simulink model "BBC"  (R2022b)
settings: Solver=VariableStepAuto  StartTime=0.0  StopTime=1  RelTol=1e-3
undefined symbols (not defined in the file): dct, dEv, Ev, sigbuilder_block
libraries: spsSeriesRLCBranchLib x3, spsVoltageMeasurementLib x2, spsControlledVoltageSourceLib x1, spsDiodeLib x1, fuzblock x1, spsGroundLib x1, spsCurrentMeasurementLib x1, spsMosfetLib x1, simulink x1, spspowerguiLib x1
settings Model: Creator=Dopechuro  LastModifiedBy=Dopechuro

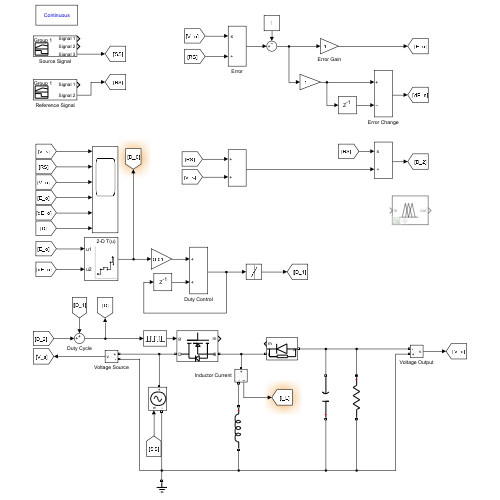
[thumbnail: Simulink's stored preview of the top-level diagram]
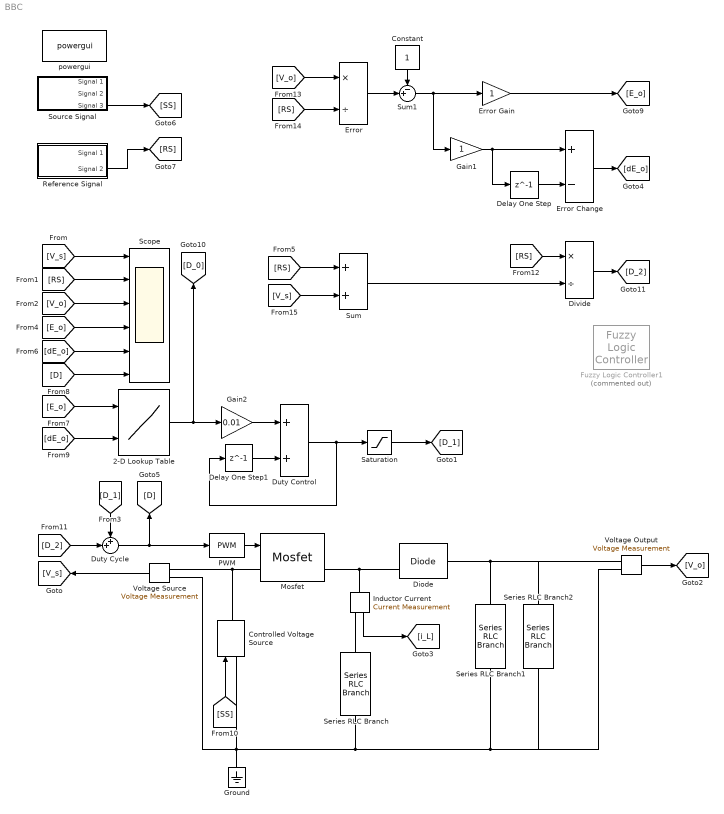
== system BBC ==
  2-D Lookup Table : Lookup_n-D  LookupTableObject=''  BreakpointsForDimension1=Ev  BreakpointsForDimension2=dEv  BreakpointsForDimension1FirstPoint=10  BreakpointsForDimension2FirstPoint=10  BreakpointsForDimension1Spacing=12  BreakpointsForDimension2Spacing=12  IndexSearchMethod=Evenly spaced points  Table=dct  InterpMethod=Nearest  DiagnosticForOutOfRangeInput=Warning  InternalRulePriority=Speed  OutDataTypeStr=Inherit: Inherit from 'Table data'  RndMeth=Simplest
      settings: InputPortMap=u0,u1
  Constant : Constant
  Controlled Voltage Source : spsControlledVoltageSourceLib/Controlled Voltage Source  Initialize=off  Source_Type=DC  Amplitude=0  Phase=0  Frequency=0  Measurements=None
  Delay One Step : Delay  DelayLength=1
  Delay One Step1 : Delay  DelayLength=1
  Diode : spsDiodeLib/Diode  Ron=0.001  Lon=0  Vf=0.8  IC=0  UseSnubber=0  Rs=500  Cs=250e-9  Measurements=on
  Divide : Product  Inputs=*/
  Duty Control : Sum
  Duty Cycle : Sum  Inputs=++|
  Error : Product  Inputs=*/
  Error Change : Sum  Inputs=+-
  Error Gain : Gain
  Fuzzy Logic Controller1 : fuzblock/Fuzzy Logic  Controller  Commented=on  FIS=bbFIS  OutputSampleNumber=101  DataType=double  FuzzifiedInputs=off  RuleFiringStrengths=off  RuleOutputs=off  AggregatedOutputs=off  SimulateUsing=Interpreted execution  OutOfRangeInputValueMessage=warning  NoRuleFiredMessage=warning  EmptyOutputFuzzySetMessage=warning
  Gain1 : Gain
  Gain2 : Gain  Gain=0.01
  Ground : spsGroundLib/Ground  LConnTagsString=a
  Inductor Current : spsCurrentMeasurementLib/Current Measurement  PhasorSimulation=off  OutputType=Complex  PSBequivalent=0
  Mosfet : spsMosfetLib/Mosfet  Ron=0.1  Lon=0  Rd=0.01  Vfd=0  IC=0  Rs=1e5  Cs=inf  Measurements=on
  PWM : simulink/Discontinuities/PWM  DisableCoverage=on  Period=1/1e5  InitialDelay=0  DisallowZeroDutyCycle=off  RunAtFixedTimeIntervals=off  SampleTime=0.1
  Reference Signal : Subsystem  Tag=STV Subsys  LoadFcn=sigbuilder_block('load');  StartFcn=sigbuilder_block('start');  StopFcn=sigbuilder_block('stop');  ClipboardFcn=sigbuilder_block('clipboard');  mask(Sigbuilder block){tuvar=[0:10]}
      mask help: Simulink:masks:SigbuilderBlock_MD
      mask init:
      | if ~strcmp(get_param(bdroot(gcbh),'SimulationStatus'),'stopped') tuvar = sigbuilder_block('maskInit'); end
      settings: CopyFcn=sigbuilder_block('copy');  DeleteFcn=sigbuilder_block('delete');  ModelCloseFcn=sigbuilder_block('modelClose');  PreSaveFcn=sigbuilder_block('preSave');  PauseFcn=sigbuilder_block('pause');  ContinueFcn=sigbuilder_block('continue');  NameChangeFcn=sigbuilder_block('namechange');  OpenFcn=sigbuilder_block('open',[530.25 309.75 550.5 399.75 ]);  CloseFcn=sigbuilder_block('close');
      mask Display: plot(0, 0, 100, 100,[2, 2, 32, 32, 2], [68, 8, 8, 68, 68],[32, 2], [38, 38], [32, 19, 2],[53, 60, 44], [32, 17, 17, 2],[16, 16, 31, 31]);txt = getActiveGroup(gcbh);text(2, 100, txt,'verticalAlignment', 'top');
  Saturation : Saturate  UpperLimit=0.9  LowerLimit=0
  Scope : Scope  NumInputPorts=6
  Series RLC Branch : spsSeriesRLCBranchLib/Series RLC Branch  LConnTagsString=__new0  RConnTagsString=__new0  BranchType=L  Resistance=1  Inductance=20e-6  SetiL0=off  InitialCurrent=0  Capacitance=1e-6  Setx0=off  InitialVoltage=0  Measurements=None
  Series RLC Branch1 : spsSeriesRLCBranchLib/Series RLC Branch  LConnTagsString=__new0  RConnTagsString=__new0  BranchType=C  Resistance=1  Inductance=1e-3  SetiL0=off  InitialCurrent=0  Capacitance=80e-6  Setx0=off  InitialVoltage=0  Measurements=None
  Series RLC Branch2 : spsSeriesRLCBranchLib/Series RLC Branch  LConnTagsString=__new0  RConnTagsString=__new0  BranchType=R  Resistance=5  Inductance=1e-3  SetiL0=off  InitialCurrent=0  Capacitance=1e-6  Setx0=off  InitialVoltage=0  Measurements=None
  Source Signal : Subsystem  Tag=STV Subsys  LoadFcn=sigbuilder_block('load');  StartFcn=sigbuilder_block('start');  StopFcn=sigbuilder_block('stop');  ClipboardFcn=sigbuilder_block('clipboard');  mask(Sigbuilder block){tuvar=[0:10]}
      mask help: Simulink:masks:SigbuilderBlock_MD
      mask init:
      | if ~strcmp(get_param(bdroot(gcbh),'SimulationStatus'),'stopped') tuvar = sigbuilder_block('maskInit'); end
      settings: CopyFcn=sigbuilder_block('copy');  DeleteFcn=sigbuilder_block('delete');  ModelCloseFcn=sigbuilder_block('modelClose');  PreSaveFcn=sigbuilder_block('preSave');  PauseFcn=sigbuilder_block('pause');  ContinueFcn=sigbuilder_block('continue');  NameChangeFcn=sigbuilder_block('namechange');  OpenFcn=sigbuilder_block('open',[395.25 256.5 550.5 399.75 ]);  CloseFcn=sigbuilder_block('close');
      mask Display: plot(0, 0, 100, 100,[2, 2, 32, 32, 2], [68, 8, 8, 68, 68],[32, 2], [38, 38], [32, 19, 2],[53, 60, 44], [32, 17, 17, 2],[16, 16, 31, 31]);txt = getActiveGroup(gcbh);text(2, 100, txt,'verticalAlignment', 'top');
  Sum : Sum
  Sum1 : Sum  Inputs=-+|
  Voltage Output : spsVoltageMeasurementLib/Voltage Measurement  PhasorSimulation=off  OutputType=Complex  PSBequivalent=0
  Voltage Source : spsVoltageMeasurementLib/Voltage Measurement  PhasorSimulation=off  OutputType=Complex  PSBequivalent=0
  powergui : spspowerguiLib/powergui  Priority=1  SimulationMode=Continuous  SampleTime=50e-6  frequency=60  Iterations=50  frequencyindice=0  Pbase=100e6  ErrMax=1e-4  UnitsV=kV  UnitsW=MW  buscounter=0  FunctionMessages=off  echomessages=off  EnableUseOfTLC=off  CurrentSourceSwitches=off  DisableSnubberDevices=off  DisableRonSwitches=off  DisableVfSwitches=off  DisplayEquations=off  AutomaticDiscreteSolvers=off  SolverType=Tustin/Backward Euler (TBE)  Interpol=off  ExternalGateDelay=off  methode=off  Ts=100  x0status=blocks  SPID=on  SwTol=0  HookPort=off  NonlinearTolerance=1e-4  nMaxIteration=100  ContinueOnMaxIteration=off  RestoreLinks=warning  ResistiveCurrentMeasurement=off  Frange=[0:2:500]  Ylog=off  Xlog=on  ShowGrid=off  save=off  variable=ZData  structure=0  ZoomFFT=off  StartTime=0.0  cycles=1  DisplayStyle=1  fundamental=60  FreqAxis=off  MaxFrequency=1000  frequencyindicesteady=1  RmsSteady=1  display=off
  wires:
  Voltage Source/1 -> [V_s]
  Inductor Current/1 -> [i_L]
  Voltage Output/1 -> [V_o]
  PWM/1 -> Mosfet/1
  [V_s] -> Scope/1
  [RS] -> Scope/2
  [V_o] -> Scope/3
  Error Change/1 -> [dE_o]
  Delay One Step/1 -> Error Change/2
  [E_o] -> Scope/4
  [dE_o] -> Scope/5
  [D] -> Scope/6
  Duty Cycle/1 -> [D], PWM/1
  [SS] -> Controlled Voltage Source/1
  [D_2] -> Duty Cycle/2
  [V_o] -> Error/1
  [RS] -> Error/2
  Error/1 -> Sum1/2
  Constant/1 -> Sum1/1
  Sum1/1 -> Gain1/1, Error Gain/1
  Error Gain/1 -> [E_o]
  Gain1/1 -> Error Change/1, Delay One Step/1
  Gain2/1 -> Duty Control/1
  Delay One Step1/1 -> Duty Control/2
  Duty Control/1 -> Saturation/1, Delay One Step1/1
  [D_1] -> Duty Cycle/1
  Saturation/1 -> [D_1]
  2-D Lookup Table/1 -> Gain2/1, [D_0]
  [E_o] -> 2-D Lookup Table/1
  [dE_o] -> 2-D Lookup Table/2
  [RS] -> Sum/1
  [V_s] -> Sum/2
  Divide/1 -> [D_2]
  Sum/1 -> Divide/2
  [RS] -> Divide/1
  Reference Signal/2(Signal 2) -> [RS]
  Source Signal/3(Signal 3) -> [SS]
  connections:
  Mosfet/LConn1 -- Controlled Voltage Source/RConn1 -- Voltage Source/LConn1
  Mosfet/RConn1 -- Inductor Current/LConn1 -- Diode/RConn1
  Diode/LConn1 -- Voltage Output/LConn2 -- Series RLC Branch2/LConn1 -- Series RLC Branch1/RConn1
  Voltage Output/LConn1 -- Series RLC Branch2/RConn1 -- Series RLC Branch1/LConn1 -- Series RLC Branch/RConn1 -- Ground/LConn1 -- Controlled Voltage Source/LConn1 -- Voltage Source/LConn2
  Inductor Current/RConn1 -- Series RLC Branch/LConn1

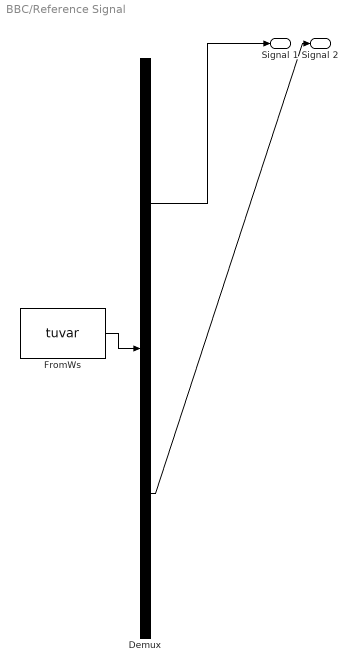
== system BBC/Reference Signal ==
  Demux : Demux  Tag=STV Demux  Outputs=2
      settings: DisplayOption=none
  FromWs : FromWorkspace  Tag=STV FromWs  VariableName=tuvar
      SigBuilderData=|
      | common.afterFinalStr = 'Extrapolate'
      | common.sampleTime = 0
      | dataSet.timeRange = [0 1]
      | dataSet.name = 'Group 1'
      | sbobj.Groups.Name = 'Group 1'
      | sbobj.Groups.Signals(1).Name = 'Signal 1'
      | sbobj.Groups.Signals(1).XData = [0 0.0111111111111 0.0222222222222 0.0333333333333 0.0444444444444 0.0555555555556 0.0666666666667 0.0777777777778 0.0888888888889 0.1 0.111111111111 0.122222222222 0.133333333333 0.144444444444 0.155555555556 0.166666666667 0.177777777778 0.188888888889 0.2 0.211111111111 0.222222222222 0.233333333333 0.244444444444 0.255555555556 0.266666666667 0.277777777778 0.288888888889 0.3 0.311111111111 0.322222222222 0.333333333333 0.344444444444 0.355555555556 0.366666666667 0.377777777778 0.388888888889 0.4 0.411111111111 0.422222222222 0.433333333333 0.444444444444 0.455555555556 0.466666666667 0.477777777778 0.488888888889 0.5 0.511111111111 0.522222222222 0.533333333333 0.544444444444 0.555555555556 0.566666666667 0.577777777778 0.588888888889 0.6 0.611111111111 0.622222222222 0.633333333333 0.644444444444 0.655555555556 0.666666666667 0.677777777778 0.688888888889 0.7 0.711111111111 0.722222222222 0.733333333333 0.744444444444 0.755555555556 0.766666666667 0.777777777778 0.788888888889 0.8 0.811111111111 0.822222222222 0.833333333333 0.844444444444 0.855555555556 0.866666666667 0.877777777778 0.888888888889 0.9 0.911111111111 0.922222222222 0.933333333333 0.944444444444 0.955555555556 0.966666666667 0.977777777778 0.988888888889 1]
      | sbobj.Groups.Signals(1).YData = [24 25.2855752194 25.969615506 25.7320508076 24.6840402867 23.3159597133 22.2679491924 22.030384494 22.7144247806 24 25.2855752194 25.969615506 25.7320508076 24.6840402867 23.3159597133 22.2679491924 22.030384494 22.7144247806 24 25.2855752194 25.969615506 25.7320508076 24.6840402867 23.3159597133 22.2679491924 22.030384494 22.7144247806 24 25.2855752194 25.969615506 25.7320508076 24.6840402867 23.3159597133 22.2679491924 22.030384494 22.7144247806 24 25.2855752194 25.969615506 25.7320508076 24.6840402867 23.3159597133 22.2679491924 22.030384494 22.7144247806 24 25.2855752194 25.969615506 25.7320508076 24.6840402867 23.3159597133 22.2679491924 22.030384494 22.7144247806 24 25.2855752194 25.969615506 25.7320508076 24.6840402867 23.3159597133 22.2679491924 22.030384494 22.7144247806 24 25.2855752194 25.969615506 25.7320508076 24.6840402867 23.3159597133 22.2679491924 22.030384494 22.7144247806 24 25.2855752194 25.969615506 25.7320508076 24.6840402867 23.3159597133 22.2679491924 22.030384494 22.7144247806 24 25.2855752194 25.969615506 25.7320508076 24.6840402867 23.3159597133 22.2679491924 22.030384494 22.7144247806 24]
      | sbobj.Groups.Signals(2).Name = 'Signal 2'
      | sbobj.Groups.Signals(2).XData = [0 0.0333333333333 0.0666666666667 0.1 0.133333333333 0.166666666667 0.2 0.233333333333 0.266666666667 0.3 0.333333333333 0.366666666667 0.4 0.433333333333 0.466666666667 0.5 0.533333333333 0.566666666667 0.6 0.633333333333 0.666666666667 0.7 0.733333333333 0.766666666667 0.8 0.833333333333 0.866666666667 0.9 0.933333333333 0.966666666667 1]
      | sbobj.Groups.Signals(2).YData = [23.2351507634 22.5977310307 22.5776240749 24.4881939099 23.8226248434 23.8039465122 25.4193101506 24.291584374 24.1978110535 25.58769909 23.1955340437 24.6966244158 24.8350881651 23.7562848596 24.2156700864 22.8341560685 22.8520472211 24.104874716 24.7222540322 26.5854912526 23.3331093293 24.1873310246 23.9175055746 22.0669770821 23.5610338461 22.2053211585 24.8403755298 23.1119679177 24.1000928331 23.45547107 24.3035207946]
      | sbobj.Groups.TimeRange = [0 1]
  Signal 1 : Outport  Tag=STV Outport
  Signal 2 : Outport  Tag=STV Outport  Port=2
  wires:
  FromWs/1 -> Demux/1
  Demux/1 -> Signal 1/1
  Demux/2 -> Signal 2/1

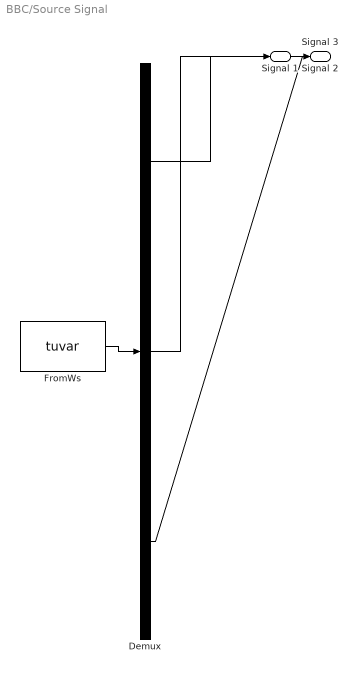
== system BBC/Source Signal ==
  Demux : Demux  Tag=STV Demux  Outputs=3
      settings: DisplayOption=none
  FromWs : FromWorkspace  Tag=STV FromWs  VariableName=tuvar
      SigBuilderData=|
      | common.afterFinalStr = 'Extrapolate'
      | common.sampleTime = 0
      | dataSet.timeRange = [0 1]
      | dataSet.name = 'Group 1'
      | sbobj.Groups.Name = 'Group 1'
      | sbobj.Groups.Signals(1).Name = 'Signal 1'
      | sbobj.Groups.Signals(1).XData = [0 1]
      | sbobj.Groups.Signals(1).YData = [24 24]
      | sbobj.Groups.Signals(2).Name = 'Signal 2'
      | sbobj.Groups.Signals(2).XData = [0 0.1 0.2 0.3 0.4 0.5 0.6 0.7 0.8 0.9 1]
      | sbobj.Groups.Signals(2).YData = [23.6998367189 24.2449826606 24.3696815618 24.8559438915 23.9029382321 22.9308223653 23.5802056263 24.677297164 23.4639223558 24.4804769349 24.0620249]
      | sbobj.Groups.Signals(3).Name = 'Signal 3'
      | sbobj.Groups.Signals(3).XData = [0 0.0222222222222 0.0444444444444 0.0666666666667 0.0888888888889 0.111111111111 0.133333333333 0.155555555556 0.177777777778 0.2 0.222222222222 0.244444444444 0.266666666667 0.288888888889 0.311111111111 0.333333333333 0.355555555556 0.377777777778 0.4 0.422222222222 0.444444444444 0.466666666667 0.488888888889 0.511111111111 0.533333333333 0.555555555556 0.577777777778 0.6 0.622222222222 0.644444444444 0.666666666667 0.688888888889 0.711111111111 0.733333333333 0.755555555556 0.777777777778 0.8 0.822222222222 0.844444444444 0.866666666667 0.888888888889 0.911111111111 0.933333333333 0.955555555556 0.977777777778 1]
      | sbobj.Groups.Signals(3).YData = [24 24.6427876097 24.984807753 24.8660254038 24.3420201433 23.6579798567 23.1339745962 23.015192247 23.3572123903 24 24.6427876097 24.984807753 24.8660254038 24.3420201433 23.6579798567 23.1339745962 23.015192247 23.3572123903 24 24.6427876097 24.984807753 24.8660254038 24.3420201433 23.6579798567 23.1339745962 23.015192247 23.3572123903 24 24.6427876097 24.984807753 24.8660254038 24.3420201433 23.6579798567 23.1339745962 23.015192247 23.3572123903 24 24.6427876097 24.984807753 24.8660254038 24.3420201433 23.6579798567 23.1339745962 23.015192247 23.3572123903 24]
      | sbobj.Groups.TimeRange = [0 1]
  Signal 1 : Outport  Tag=STV Outport
  Signal 2 : Outport  Tag=STV Outport  Port=2
  Signal 3 : Outport  Tag=STV Outport  Port=3
  wires:
  FromWs/1 -> Demux/1
  Demux/1 -> Signal 1/1
  Demux/2 -> Signal 2/1
  Demux/3 -> Signal 3/1
